simulink model "MBKwithLQDG_TCACS"  (R2020a)
settings: Solver=ode4  StartTime=0.0  StopTime=20  FixedStep=0.01  RelTol=1e-3
InitFcn:
  | MBK
values from neighbouring files (symbols this model uses):
  b = [100, 100,   20]    [Finder.m]
undefined symbols (not defined in the file or in its folder): k, m, X
settings Model: Creator=Ali  LastModifiedBy=Ali
settings DataIOCC: ReturnWorkspaceOutputs=off
settings DebuggingCC: ArithmeticOperatorsInVariantConditions=warning
settings SFSimCC: SimUseLocalCustomCode=off  CustomCodeUndefinedFunction=UseInterfaceOnly
settings RTWCC: RTWUseLocalCustomCode=off

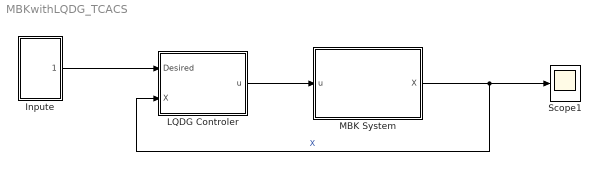
== system MBKwithLQDG_TCACS ==
  Inpute : Subsystem
  LQDG Controler : Subsystem
  MBK System : Subsystem
  Scope1 : Scope
  wires:
  MBK System/1(X) -> LQDG Controler/2(X), Scope1/1  "X"
  LQDG Controler/1(u) -> MBK System/1(u)
  Inpute/1(Desired) -> LQDG Controler/1(Desired)

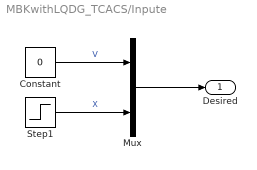
== system MBKwithLQDG_TCACS/Inpute ==
  Constant : Constant  Value=0
  Mux : Mux  Inputs=2
  Step1 : Step  After=6  SampleTime=0
  Desired : Outport  VectorParamsAs1DForOutWhenUnconnected=off
  wires:
  Mux/1 -> Desired/1
  Step1/1 -> Mux/2  "X"
  Constant/1 -> Mux/1  "V"

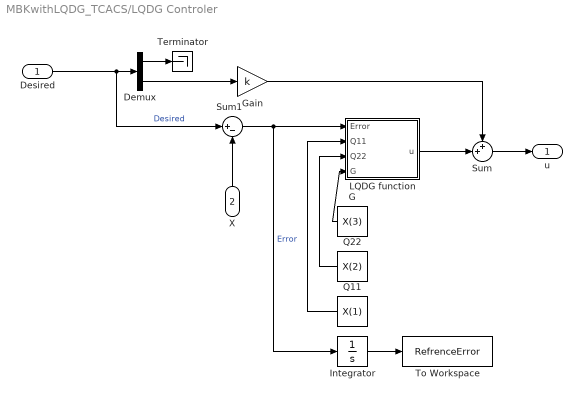
== system MBKwithLQDG_TCACS/LQDG Controler ==
  Desired : Inport
  X : Inport  Port=2
  Demux : Demux  Outputs=2
  G : Constant  Value=X(3)
  Gain : Gain  Gain=k
  Integrator : Integrator
  LQDG function : MATLAB Function  TreatAsAtomicUnit=on
  Q11 : Constant  Value=X(1)
  Q22 : Constant  Value=X(2)
  Sum : Sum  Inputs=++|
  Sum1 : Sum  Inputs=|+-
  Terminator : Terminator
  To Workspace : ToWorkspace  VariableName=RefrenceError  SampleTime=-1
      settings: Save2DSignal=2-D array (concatenate along first dimension)
  u : Outport  VectorParamsAs1DForOutWhenUnconnected=off
  wires:
  X/1 -> Sum1/2
  LQDG function/1(u) -> Sum/2
  Sum/1 -> u/1
  Gain/1 -> Sum/1
  Desired/1 -> Sum1/1, Demux/1  "Desired"
  Demux/2 -> Gain/1
  Demux/1 -> Terminator/1
  G/1 -> LQDG function/4(G)
  Q22/1 -> LQDG function/3(Q22)
  Q11/1 -> LQDG function/2(Q11)
  Integrator/1 -> To Workspace/1
  Sum1/1 -> Integrator/1, LQDG function/1(Error)  "Error"

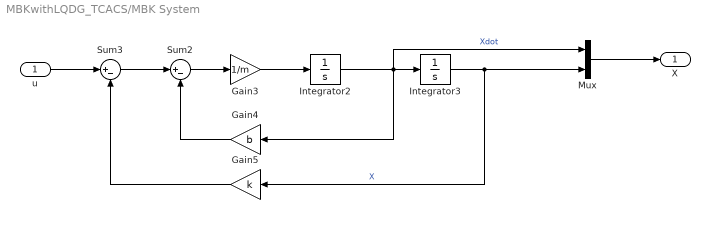
== system MBKwithLQDG_TCACS/MBK System ==
  u : Inport
  Gain3 : Gain  Gain=1/m
  Gain4 : Gain  Gain=b
  Gain5 : Gain  Gain=k
  Integrator2 : Integrator
  Integrator3 : Integrator  InitialCondition=3
  Mux : Mux  Inputs=2
  Sum2 : Sum  Inputs=|+-
  Sum3 : Sum  Inputs=|+-
  X : Outport  VectorParamsAs1DForOutWhenUnconnected=off
  wires:
  u/1 -> Sum3/1
  Gain4/1 -> Sum2/2
  Gain3/1 -> Integrator2/1
  Integrator3/1 -> Mux/2, Gain5/1  "X"
  Gain5/1 -> Sum3/2
  Sum2/1 -> Gain3/1
  Integrator2/1 -> Mux/1, Gain4/1, Integrator3/1  "Xdot"
  Sum3/1 -> Sum2/1
  Mux/1 -> X/1

== matlab function MBKwithLQDG_TCACS/LQDG Controler/LQDG function ==
  settings: updateMethod=DISCRETE
  data: u output; Error input; Q11 input; Q22 input; G input
function u = LQDG(Error, Q11, Q22, G)
%% System Description
% Mass
m = 10;
% Viscous Friction Coefficient 
b = 2;
% Spring Constant
k = 5;
%% State Space
% x_dot = Ax + Bu - Dv (DV: Disturbance)

A = [ 0    1;
    -k/m -b/m];
%C = [0 1];
B = [ 0 ;
     1/m];
D = B;
% Weight Matrix
R = 1;
Q = [Q11 0;
     0   Q22] ;
%G = 2;
%% Riccati Equation
persistent Forloop;
persistent P_ans;
if isempty(Forloop) % use for simulink
    Forloop = 0;
    P_ans = zeros(2, 2);
    P12   = zeros(1, 2);
    % P * A + A' * P - P * B * R^-1 * B' * P + P * D * G^-1 * D' * P + Q
    % first equation Q(1, 1) - P12^2/m^2 + P12^2/(G*m^2) - (2*P12*k)/m = 0
    % Ans1 P12 = -(G*m*(k - ((G*k^2 - Q(1, 1) + G*Q(1, 1))/G)^(1/2)))/(G - 1)
    % Ans2 P12 = -(G*m*(k - ((G*k^2 - Q(1, 1) + G*Q(1, 1))/G)^(1/2)))/(G - 1)
    if ((G*k^2 - Q(1, 1) + G*Q(1, 1))/G) >= 0
        P12(1) = -(G*m*(k - ((G*k^2 - Q(1, 1) + G*Q(1, 1))/G)^(1/2)))/(G - 1);
        P12(2) = -(G*m*(k - ((G*k^2 - Q(1, 1) + G*Q(1, 1))/G)^(1/2)))/(G - 1);
    else
        P12(1) = Inf;
        P12(2) = Inf;
    end
    for i = 1:length(P12)
        if P12(i) == Inf
            continue;
        end
        % Second equation 2*P12 + Q(2, 2) - P22^2/m^2 + P22^2/(G*m^2) -
        % (2*P22*b)/m = 0
        % Ans1 K12 =  -(G*m*(b + ((G*b^2 - 2*P12 - Q(2, 2) + 2*G*P12 + G*Q(2, 2))/G)^(1/2)))/(G - 1)
        % Ans2 K12 =  -(G*m*(b - ((G*b^2 - 2*P12 - Q(2, 2) + 2*G*P12 + G*Q(2, 2))/G)^(1/2)))/(G - 1)
        P22 = zeros(1, 2);
        if ((G*b^2 - 2*P12(i) - Q(2, 2) + 2*G*P12(i) + G*Q(2, 2))/G) >= 0
            P22(1) = -(G*m*(b + ((G*b^2 - 2*P12(i) - Q(2, 2) + 2*G*P12(i) + G*Q(2, 2))/G)^(1/2)))/(G - 1);
            P22(2) = -(G*m*(b - ((G*b^2 - 2*P12(i) - Q(2, 2) + 2*G*P12(i) + G*Q(2, 2))/G)^(1/2)))/(G - 1);
        else
            P22(2) = Inf;
            P22(1) = Inf;
        end
        for j = 1:length(P22)
            if P22(j) == Inf
                continue
            end
            % Last equation P11 - (P12*P22)/m^2 - (P12*b)/m - (P22*k)/m + (P12*P22)/(G*m^2)
            % Ans P11 = (P12*P22)/m^2 + (P12*b)/m + (P22*k)/m - (P12*P22)/(G*m^2)
            P11 = (P12(i)*P22(j) + P12(i)*b*m + P22(j)*k*m)/m^2;
            temp_P = zeros(2, 2);
            temp_P(1, 1) = P11;
            temp_P(1, 2) = P12(i);
            temp_P(2, 1) = P12(i);
            temp_P(2, 2) = P22(j);
            if all(eig(A - B * R^(-1)* B' * temp_P + D * G^-1 * D' * temp_P ) < 0)
                Forloop = 1;
                P_ans = temp_P;
                break;
            end
        end
        if Forloop == 1
            break;
        end
    end
end
u = (R^-1)*B'*P_ans*Error;
